simulink model "Bio_batch"  (R2022a)
settings: Solver=ode15s  StartTime=0.0  StopTime=24.1  RelTol=1e-4  AbsTol=1e-4
settings Model: SimulationMode=accelerator  Creator=César-Garech  LastModifiedBy=DELL
settings SolverCC: AlgebraicLoopSolver=TrustRegion  SolverResetMethod=Robust
settings DataIOCC: SaveFormat=Array  ReturnWorkspaceOutputs=off
settings DebuggingCC: UnconnectedInputMsg=warning  UnconnectedOutputMsg=warning  UnconnectedLineMsg=warning  SFMachineParentedDataDiag=warning
settings RTWCC: DLArmComputeVersion=19.05

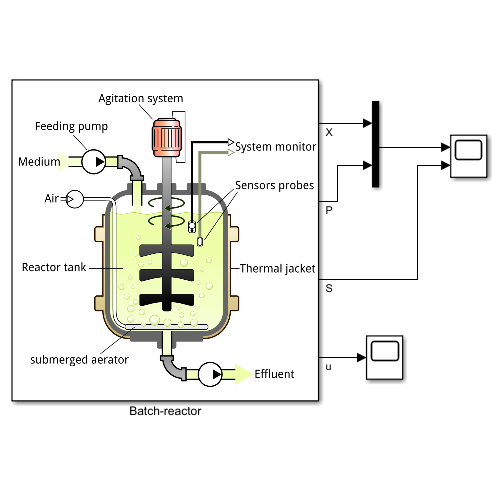
[thumbnail: Simulink's stored preview of the top-level diagram]
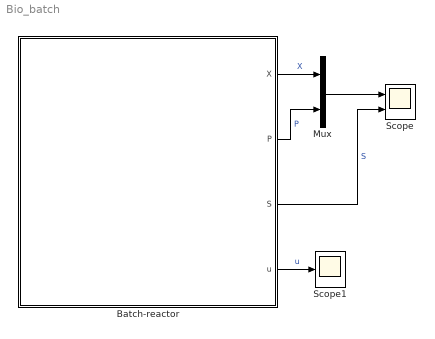
== system Bio_batch ==
  Batch-reactor : Subsystem
      mask Display: image('biorreactor.png'); % Use "Edit Image" on toolstrip to change.
  Mux : Mux  Inputs=2
  Scope : Scope  NumInputPorts=2
  Scope1 : Scope
  wires:
  Mux/1 -> Scope/1
  Batch-reactor/1(X) -> Mux/1  "X"
  Batch-reactor/2(P) -> Mux/2  "P"
  Batch-reactor/4(u) -> Scope1/1  "u"
  Batch-reactor/3(S) -> Scope/2  "S"

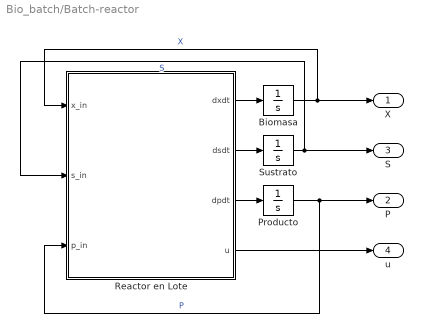
== system Bio_batch/Batch-reactor ==
  Biomasa : Integrator  InitialCondition=1.0976
  Producto : Integrator
  Reactor en Lote : MATLAB Function  TreatAsAtomicUnit=on
  Sustrato : Integrator  InitialCondition=84.6948
  X : Outport
  P : Outport  Port=2
  S : Outport  Port=3
  u : Outport  Port=4
  wires:
  Reactor en Lote/3(dpdt) -> Producto/1
  Biomasa/1 -> X/1, Reactor en Lote/1(x_in)  "X"
  Producto/1 -> Reactor en Lote/3(p_in), P/1  "P"
  Reactor en Lote/2(dsdt) -> Sustrato/1
  Reactor en Lote/1(dxdt) -> Biomasa/1
  Sustrato/1 -> S/1, Reactor en Lote/2(s_in)  "S"
  Reactor en Lote/4(u) -> u/1

== matlab function Bio_batch/Batch-reactor/Reactor en Lote ==
  data: x_in input; dxdt output; s_in input; p_in input; dsdt output; dpdt output; u output
function [dxdt, dsdt,dpdt,u] =Bio_batch(x_in,s_in,p_in)

%Definir Parámetros
Optim=[0.435603540944362,0.642245439116729,1.68836415295721,2.62700396764849,1.83188078300514,99.9928951768216,99.9948789027871];

umax=0.85*Optim(1);
Yxs=0.8*Optim(2);
Ks=0.08*Optim(3);
alfa=0.05*Optim(4);
beta=0.002*Optim(5);
Smax=90*Optim(6);
ms=0.00001*Optim(7);


%Condiciones iniciales
x=x_in;
s=s_in;
p=p_in;

%Ecuaciones constitutivas
u=umax*(s/(Ks+s)*(1-(s/Smax))); %h^-1
Rx=u*x;
Rs=(u/(Yxs)+ms)*x;
Rp=(alfa*u+beta)*x;

%Balances
dxdt=Rx;
dsdt=-Rs;
dpdt=Rp;

end
